simulink model "CurtisEnable"  (R2024a)
settings: Solver=FixedStepAuto  StartTime=0.0  StopTime=20  RelTol=1e-3
model workspace (MAT data in the model file):
  mdlWSDbList = ["tramontina_database_curtis.dbc" "tramontina_database_curtis_mesa.dbc"]
undefined symbols (not defined in the file): Down, Pull
libraries: tramontina_database_curtislib x5, tramontina_database_curtis_mesalib x4, speedgoatlib_IO60X_IO69X x3, speedgoatlib_IO691 x1
settings Model: Creator=anderson.bordin  LastModifiedBy=matlab.cut
settings SolverCC: ConcurrentTasks=on  PositivePriorityOrder=on
settings OptimizationCC: BlockReduction=off  OptimizeBlockIOStorage=off  EnhancedBackFolding=on  PassReuseOutputArgsThreshold=0  MaxStackSize=64  OptimizeBlockOrder=speed  DifferentSizesBufferReuse=on
settings DebuggingCC: TasksWithSamePriorityMsg=none  ParameterTunabilityLossMsg=error
settings HardwareCC: ProdBitPerLong=64  ProdLongLongMode=on  ProdHWDeviceType=Intel->x86-64 (Linux 64)
settings SFSimCC: MATLABDynamicMemAlloc=off
settings RTWCC: Description=Speedgoat Real-Time Target Machine  SystemTargetFile=speedgoat.tlc  TemplateMakefile=slrealtime_default_tmf  Toolchain=Simulink Real-Time Toolchain  BuildConfiguration=Faster Runs  CodeExecutionProfiling=on  TargetLang=C++
settings CodeAppCC: ForceParamTrailComments=on  OperatorAnnotations=on
settings SimulinkRealTimeTargetCC: InstructionSetFMA=off  LogToMDFFile=off

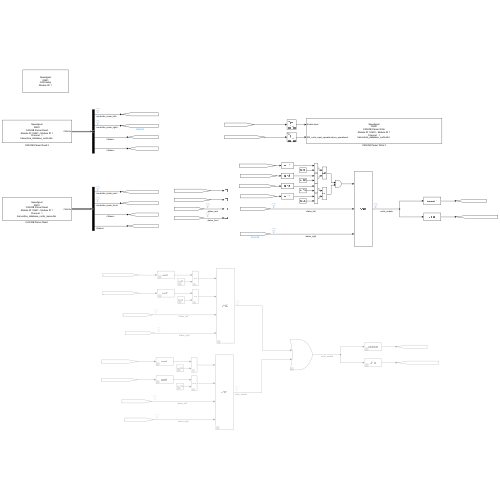
[thumbnail: Simulink's stored preview of the top-level diagram]
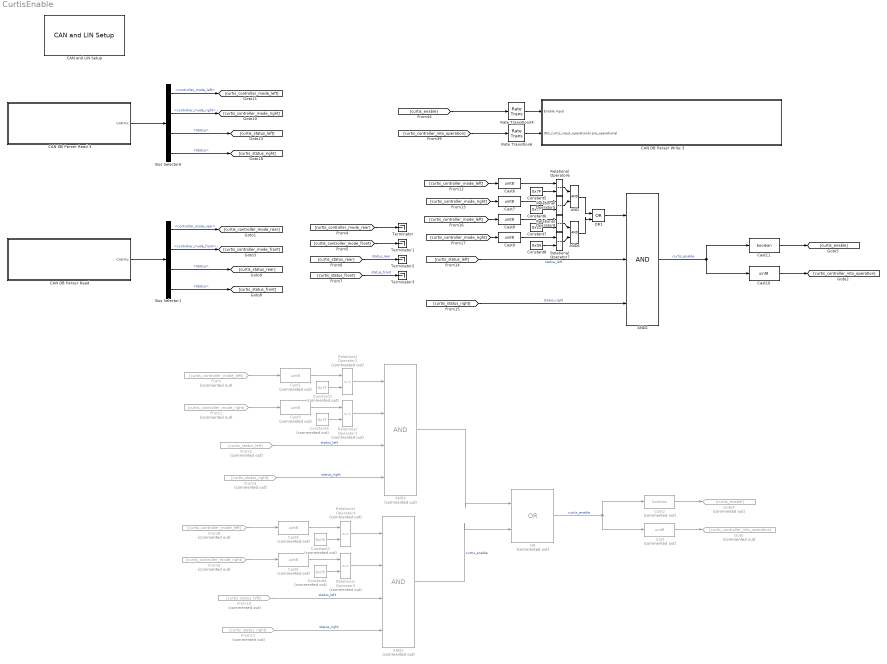
== system CurtisEnable ==
  AND : Logic  AllPortsSameDT=off  OutDataTypeStr=boolean
  AND1 : Logic  Commented=on  Inputs=4  AllPortsSameDT=off  OutDataTypeStr=boolean
  AND2 : Logic  Inputs=3  AllPortsSameDT=off  OutDataTypeStr=boolean
  AND3 : Logic  Commented=on  Inputs=4  AllPortsSameDT=off  OutDataTypeStr=boolean
  AND4 : Logic  AllPortsSameDT=off  OutDataTypeStr=boolean
  Bus Selector1 : BusSelector  OutputSignals=ID1833_controller_status_RCUrear.controller_mode_rear,ID1832_controller_status_RCUfront.controller_mode_front,ID425_curtis_feedback_message_RCUrear.MessageStatus.Status,ID424_curtis_feedback_message_RCUfront.MessageStatus.Status
  Bus Selector6 : BusSelector  OutputSignals=ID1830_controller_status_left.controller_mode_left,ID1831_controller_status_right.controller_mode_right,ID1830_controller_status_left.MessageStatus.Status,ID1831_controller_status_right.MessageStatus.Status
  "CAN DB Parser Read " : Subsystem
      settings: OpenFcn=sg_can.OpenFcnRead;
      mask Help: eval('sg.utils.help.show(''io_main/refentry_ref_can_ofa_parsing_read'');')
      mask Display: disp('Speedgoat\nIO691\nCAN DB Parser Read\nModule ID: IO691 - Module ID 1\nChannel:  1\ntramontina_database_curtis_mesa.dbc ');
  CAN DB Parser Read 3 : Subsystem
      settings: OpenFcn=sg_can.OpenFcnRead;
      mask Help: eval('sg.utils.help.show(''io_main/refentry_ref_can_ofa_parsing_read'');')
      mask Display: disp('Speedgoat\nIO691\nCAN DB Parser Read\nModule ID: IO691 - Module ID 1\nChannel:  1\ntramontina_database_curtis.dbc ');
  CAN DB Parser Write 3 : Subsystem
      settings: OpenFcn=sg_can.OpenFcnWrite;
      mask Help: eval('sg.utils.help.show(''io_main/refentry_ref_can_ofa_parsing_write'');')
      mask Display: disp('Speedgoat\nIO691\nCAN DB Parser Write\nModule ID: IO691 - Module ID 1\nChannel:  1\ntramontina_database_curtis.dbc ');
  "CAN and LIN Setup " : speedgoatlib_IO691/CAN and LIN Setup   moduleInitValues="[691    1    1   -1   -1]"  id=1  moduleType=IO691  pciSlot=-1  canChn1=CAN (HS)  canChn2=Disabled  canChn3=Disabled  canChn4=Disabled  linChn1=Disabled  linChn2=Disabled  canInitStructArray=[]  canTermStructArray=[]  gpioChnx=Disabled  canChn1InitValues="[2   2   8   1  16   3  19   2   2   5   2   0]"  arbBdrChn1=500 kBaud  clockDividerChn1=Enable  arbManBdrChn1=[8,1,16,3]  fdBdrChn1=5.0 MBaud  fdManBdrChn1=[2,2,5,2]  termResistor1=off  canChn2InitValues="[1   0   2   8  31   8  19   2   2   5   2   0]"  arbBdrChn2=1.0 MBaud  clockDividerChn2=Enable  arbManBdrChn2=[2,8,31,8]  fdBdrChn2=5.0 MBaud  fdManBdrChn2=[2,2,5,2]  termResistor2=off  canChn3InitValues="[1   0   2   8  31   8  19   2   2   5   2   0]"  arbBdrChn3=1.0 MBaud  clockDividerChn3=Enable  arbManBdrChn3=[2,8,31,8]  fdBdrChn3=5.0 MBaud  fdManBdrChn3=[2,2,5,2]  termResistor3=off  canChn4InitValues="[1   0   2   8  31   8  19   2   2   5   2   0]"  arbBdrChn4=1.0 MBaud  clockDividerChn4=Enable  arbManBdrChn4=[2,8,31,8]  fdBdrChn4=5.0 MBaud  fdManBdrChn4=[2,2,5,2]  termResistor4=off  linChn1InitValues="[0  9600]"  linBtrChn1=9600  linChn2InitValues="[0  9600]"  linBtrChn2=9600  doInitTermStruct="[0  5  0  0  0]"  parDoChannels=[1 2]  parDoVoltage=5  parDoInitValues=0  parDoReset=1  parNumOfDoS=0  parDiChannels=[3 4]  parDiVoltage=5  parDiPull=Pull-Down
      settings: LibrarySourceBlock=speedgoatlib_IO602_IO691/CAN and LIN Setup
  Cast{,1,3..5} (5 alike) : DataTypeConversion  Commented=on  OutDataTypeStr=uint8  SaturateOnIntegerOverflow=off  RndMeth=Floor
  Cast{6..10} (5 alike) : DataTypeConversion  OutDataTypeStr=uint8  SaturateOnIntegerOverflow=off  RndMeth=Floor
  Cast11 : DataTypeConversion  OutDataTypeStr=boolean  SaturateOnIntegerOverflow=off  RndMeth=Floor
  Cast2 : DataTypeConversion  Commented=on  OutDataTypeStr=boolean  SaturateOnIntegerOverflow=off  RndMeth=Floor
  Constant1 : Constant  Commented=on  Value=0x05
  Constant2 : Constant  Commented=on  Value=0x7F
  Constant3 : Constant  Commented=on  Value=0x7F
  Constant4 : Constant  Commented=on  Value=0x05
  Constant5 : Constant  Value=0x7F
  Constant6 : Constant  Value=0x7F
  Constant7 : Constant  Value=0x05
  Constant8 : Constant  Value=0x05
  From : From  Commented=on  GotoTag=curtis_controller_mode_left
  From1 : From  Commented=on  GotoTag=curtis_controller_mode_right
  From10 : From  Commented=on  GotoTag=curtis_status_left
  From11 : From  Commented=on  GotoTag=curtis_status_right
  From2 : From  Commented=on  GotoTag=curtis_status_left
  From3 : From  Commented=on  GotoTag=curtis_status_right
  From8 : From  Commented=on  GotoTag=curtis_controller_mode_left
  From9 : From  Commented=on  GotoTag=curtis_controller_mode_right
  Goto : Goto  Commented=on  GotoTag=curtis_controller_into_operation
  Goto4 : Goto  Commented=on  GotoTag=curtis_enable
  OR : Logic  Commented=on  Operator=OR  IconShape=distinctive  AllPortsSameDT=off  OutDataTypeStr=boolean
  OR1 : Logic  Operator=OR  IconShape=distinctive  AllPortsSameDT=off  OutDataTypeStr=boolean
  Rate Transition24 : RateTransition
  Rate Transition6 : RateTransition
  Relational Operator{1..4} (4 alike) : RelationalOperator  Commented=on  Operator===  OutDataTypeStr=boolean  RndMeth=Simplest  InputSameDT=off
  Relational Operator{5..8} (4 alike) : RelationalOperator  Operator===  OutDataTypeStr=boolean  RndMeth=Simplest  InputSameDT=off
  Terminator{,1..3} (4 alike) : Terminator
  wires:
  Relational Operator1/1 -> AND3/2
  From/1 -> Cast1/1
  Constant3/1 -> Relational Operator1/2
  From3/1 -> AND3/4  "status_right"
  From2/1 -> AND3/3  "status_left"
  From1/1 -> Cast3/1
  Cast/1 -> Goto/1
  Cast2/1 -> Goto4/1
  Constant2/1 -> Relational Operator2/2
  Cast3/1 -> Relational Operator1/1
  Relational Operator2/1 -> AND3/1
  Cast1/1 -> Relational Operator2/1
  Bus Selector6/1 -> [curtis_controller_mode_left]  "<controller_mode_left>"
  CAN DB Parser Read 3/1(CAN Rx) -> Bus Selector6/1
  Bus Selector6/2 -> [curtis_controller_mode_right]  "<controller_mode_right>"
  Bus Selector6/3 -> [curtis_status_left]  "<Status>"
  Bus Selector6/4 -> [curtis_status_right]  "<Status>"
  [curtis_controller_into_operation] -> Rate Transition6/1
  Rate Transition6/1 -> CAN DB Parser Write 3/2(ID0_curtis_input_operational.pre_operational)
  [curtis_enable] -> Rate Transition24/1
  Bus Selector1/1 -> [curtis_controller_mode_rear]  "<controller_mode_rear>"
  Bus Selector1/2 -> [curtis_controller_mode_front]  "<controller_mode_front>"
  "CAN DB Parser Read "/1(CAN Rx) -> Bus Selector1/1
  Bus Selector1/4 -> [curtis_status_front]  "<Status>"
  Bus Selector1/3 -> [curtis_status_rear]  "<Status>"
  [curtis_controller_mode_rear] -> Terminator/1
  [curtis_controller_mode_front] -> Terminator1/1
  [curtis_status_rear] -> Terminator2/1  "status_rear"
  [curtis_status_front] -> Terminator3/1  "status_front"
  Rate Transition24/1 -> CAN DB Parser Write 3/1(Enable Input)
  Cast4/1 -> Relational Operator4/1
  Relational Operator4/1 -> AND1/1
  Cast5/1 -> Relational Operator3/1
  Constant1/1 -> Relational Operator4/2
  From9/1 -> Cast5/1
  From10/1 -> AND1/3  "status_left"
  From11/1 -> AND1/4  "status_right"
  Constant4/1 -> Relational Operator3/2
  From8/1 -> Cast4/1
  Relational Operator3/1 -> AND1/2
  AND3/1 -> OR/1
  AND1/1 -> OR/2  "curtis_enable"
  OR/1 -> Cast/1, Cast2/1  "curtis_enable"
  Cast6/1 -> Relational Operator6/1
  Cast7/1 -> Relational Operator5/1
  Constant5/1 -> Relational Operator6/2
  [curtis_controller_mode_right] -> Cast7/1
  [curtis_status_left] -> AND2/2  "status_left"
  [curtis_status_right] -> AND2/3  "status_right"
  Constant6/1 -> Relational Operator5/2
  [curtis_controller_mode_left] -> Cast6/1
  Relational Operator6/1 -> AND/1
  Relational Operator5/1 -> AND/2
  Relational Operator7/1 -> AND4/2
  Relational Operator8/1 -> AND4/1
  [curtis_controller_mode_left] -> Cast8/1
  Constant8/1 -> Relational Operator7/2
  [curtis_controller_mode_right] -> Cast9/1
  Constant7/1 -> Relational Operator8/2
  Cast9/1 -> Relational Operator7/1
  Cast8/1 -> Relational Operator8/1
  AND/1 -> OR1/1
  AND4/1 -> OR1/2
  OR1/1 -> AND2/1
  AND2/1 -> Cast11/1, Cast10/1  "curtis_enable"
  Cast11/1 -> [curtis_enable]
  Cast10/1 -> [curtis_controller_into_operation]

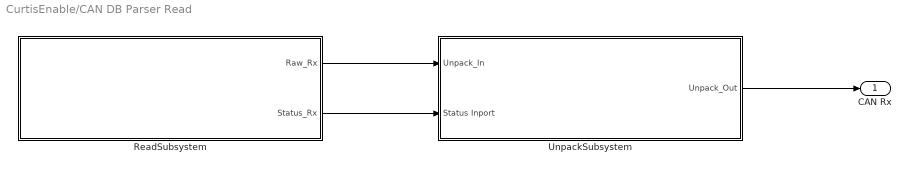
== system CurtisEnable/CAN DB Parser Read  ==
  ReadSubsystem : Subsystem
  UnpackSubsystem : Subsystem
  CAN Rx : Outport
  wires:
  ReadSubsystem/1(Raw_Rx) -> UnpackSubsystem/1(Unpack_In)
  ReadSubsystem/2(Status_Rx) -> UnpackSubsystem/2(Status Inport)
  UnpackSubsystem/1(Unpack_Out) -> CAN Rx/1

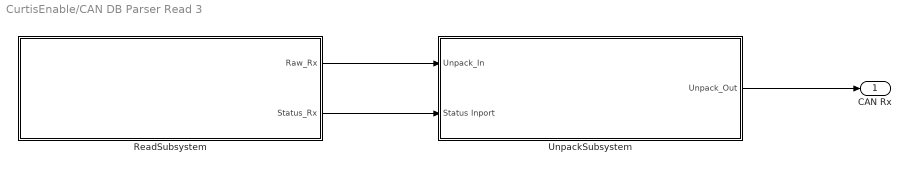
== system CurtisEnable/CAN DB Parser Read 3 ==
  ReadSubsystem : Subsystem
  UnpackSubsystem : Subsystem
  CAN Rx : Outport
  wires:
  ReadSubsystem/1(Raw_Rx) -> UnpackSubsystem/1(Unpack_In)
  ReadSubsystem/2(Status_Rx) -> UnpackSubsystem/2(Status Inport)
  UnpackSubsystem/1(Unpack_Out) -> CAN Rx/1

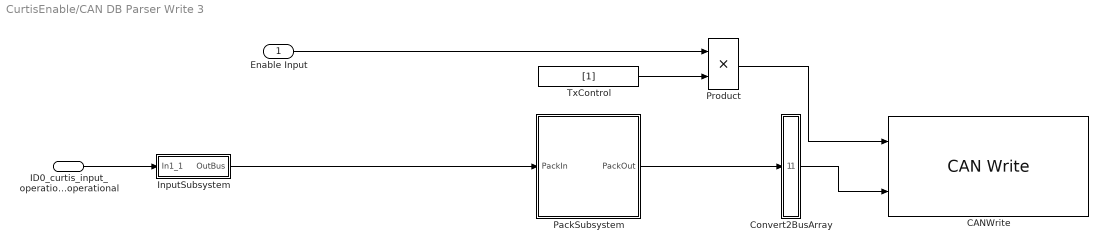
== system CurtisEnable/CAN DB Parser Write 3 ==
  Enable Input : Inport  OutDataTypeStr=boolean
  ID0_curtis_input_operational.pre_operational : Inport  Port=2
  CANWrite : speedgoatlib_IO60X_IO69X/CAN/CAN Write   moduleType=IO691  id=1  channel=1  canType=CAN (HS)  messageType=CAN (HS)  useBusIn=on  numOfMsg=1  enableInput=on  enableStatusPort=off  ts=500e-3  initValues=[691 1 0.5 0 1 1 0 1 1 1]
  Convert2BusArray : Subsystem
  InputSubsystem : Subsystem
  PackSubsystem : Subsystem
  Product : Product  OutDataTypeStr=uint32
  TxControl : Constant  Value=[1]  OutDataTypeStr=uint32
  wires:
  PackSubsystem/1(PackOut) -> Convert2BusArray/1(InBus)
  Convert2BusArray/1(BusArrayOut) -> CANWrite/2
  Product/1 -> CANWrite/1
  TxControl/1 -> Product/2
  Enable Input/1 -> Product/1
  ID0_curtis_input_operational.pre_operational/1 -> InputSubsystem/1(In1_1)
  InputSubsystem/1(OutBus) -> PackSubsystem/1(PackIn)

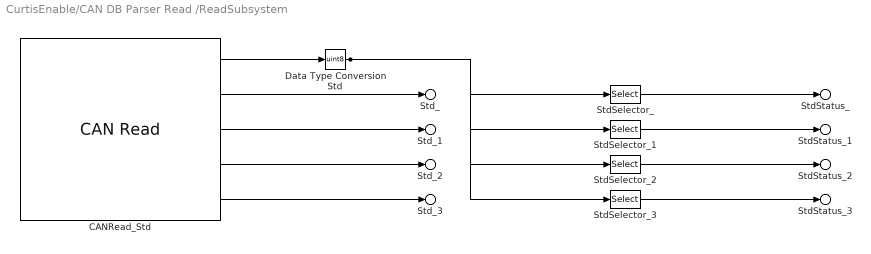
== system CurtisEnable/CAN DB Parser Read /ReadSubsystem ==
  CANRead_Std : speedgoatlib_IO60X_IO69X/CAN/CAN Read   moduleType=IO691  id=1  channel=1  canType=CAN (HS)  messageType=CAN (HS)  useBusOut=on  HasMulRead=Specify by IDs  MsgIDlist="[424   425  1832  1833]"  isEFF=off  LabelInHex=off  enableInput=off  initValues=[691 1 0.05 0 1 1 0 1 2 0 4 424 425 1832 1833]  ts=50e-3
  Data Type ConversionStd : DataTypeConversion  OutDataTypeStr=uint8  SaturateOnIntegerOverflow=off  RndMeth=Floor
  StdSelector_ : Selector  IndexOptions=Index vector (dialog)  Indices=1  OutputSizes=1
  StdSelector_1 : Selector  IndexOptions=Index vector (dialog)  Indices=2  OutputSizes=1
  StdSelector_2 : Selector  IndexOptions=Index vector (dialog)  Indices=3  OutputSizes=1
  StdSelector_3 : Selector  IndexOptions=Index vector (dialog)  Indices=4  OutputSizes=1
  Std_ : Outport  PortName=Raw_Rx  Element=Std.ID424
  Std_1 : Outport  PortName=Raw_Rx  Element=Std.ID425
  Std_2 : Outport  PortName=Raw_Rx  Element=Std.ID1832
  Std_3 : Outport  PortName=Raw_Rx  Element=Std.ID1833
  StdStatus_ : Outport  Port=2  PortName=Status_Rx  Element=Std.ID424
  StdStatus_1 : Outport  Port=2  PortName=Status_Rx  Element=Std.ID425
  StdStatus_2 : Outport  Port=2  PortName=Status_Rx  Element=Std.ID1832
  StdStatus_3 : Outport  Port=2  PortName=Status_Rx  Element=Std.ID1833
  wires:
  CANRead_Std/1 -> Data Type ConversionStd/1
  CANRead_Std/2 -> Std_/1
  CANRead_Std/3 -> Std_1/1
  CANRead_Std/4 -> Std_2/1
  CANRead_Std/5 -> Std_3/1
  Data Type ConversionStd/1 -> StdSelector_/1, StdSelector_1/1, StdSelector_2/1, StdSelector_3/1
  StdSelector_/1 -> StdStatus_/1
  StdSelector_1/1 -> StdStatus_1/1
  StdSelector_2/1 -> StdStatus_2/1
  StdSelector_3/1 -> StdStatus_3/1

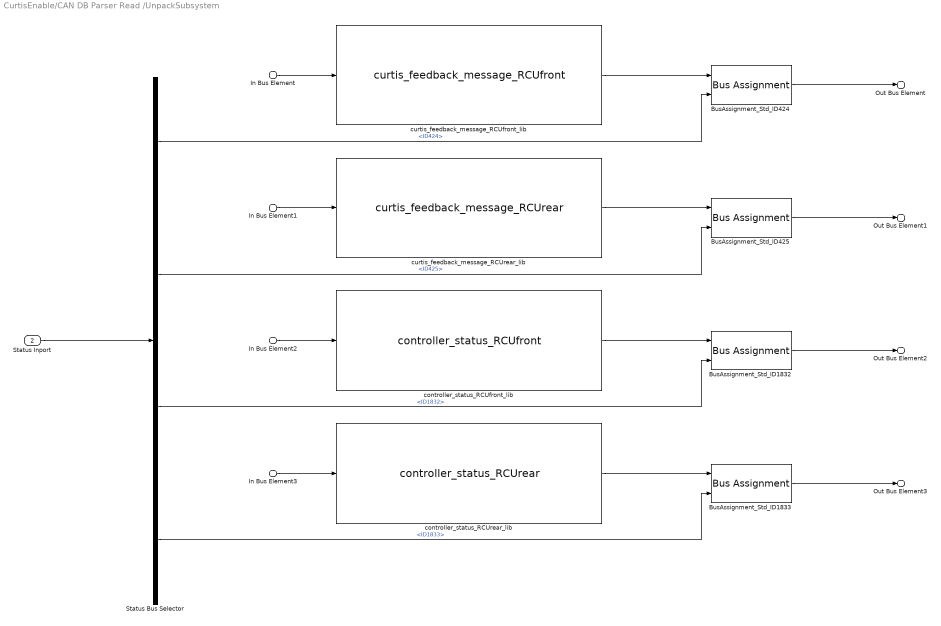
== system CurtisEnable/CAN DB Parser Read /UnpackSubsystem ==
  In Bus Element : Inport  PortName=Unpack_In  Element=Std.ID424
  In Bus Element1 : Inport  PortName=Unpack_In  Element=Std.ID425
  In Bus Element2 : Inport  PortName=Unpack_In  Element=Std.ID1832
  In Bus Element3 : Inport  PortName=Unpack_In  Element=Std.ID1833
  Status Inport : Inport  Port=2
  BusAssignment_Std_ID{424..425,1832..1833} (4 alike) : BusAssignment  AssignedSignals=MessageStatus.Status
  Status Bus Selector : BusSelector  OutputSignals=Std.ID424,Std.ID425,Std.ID1832,Std.ID1833
  controller_status_RCUfront_lib : tramontina_database_curtis_mesalib/CAN unpack/controller_status_RCUfront  SystemSampleTime=-1  VariantActivationTime=update diagram  AllowFlexibleInterface=on  Latency=0  AutoFrameSizeCalculation=off
  controller_status_RCUrear_lib : tramontina_database_curtis_mesalib/CAN unpack/controller_status_RCUrear  SystemSampleTime=-1  VariantActivationTime=update diagram  AllowFlexibleInterface=on  Latency=0  AutoFrameSizeCalculation=off
  curtis_feedback_message_RCUfront_lib : tramontina_database_curtis_mesalib/CAN unpack/curtis_feedback_message_RCUfront  SystemSampleTime=-1  VariantActivationTime=update diagram  AllowFlexibleInterface=on  Latency=0  AutoFrameSizeCalculation=off
  curtis_feedback_message_RCUrear_lib : tramontina_database_curtis_mesalib/CAN unpack/curtis_feedback_message_RCUrear  SystemSampleTime=-1  VariantActivationTime=update diagram  AllowFlexibleInterface=on  Latency=0  AutoFrameSizeCalculation=off
  Out Bus Element : Outport  PortName=Unpack_Out  Element=ID424_curtis_feedback_message_RCUfront
  Out Bus Element1 : Outport  PortName=Unpack_Out  Element=ID425_curtis_feedback_message_RCUrear
  Out Bus Element2 : Outport  PortName=Unpack_Out  Element=ID1832_controller_status_RCUfront
  Out Bus Element3 : Outport  PortName=Unpack_Out  Element=ID1833_controller_status_RCUrear
  wires:
  In Bus Element/1 -> curtis_feedback_message_RCUfront_lib/1
  curtis_feedback_message_RCUfront_lib/1 -> BusAssignment_Std_ID424/1
  BusAssignment_Std_ID424/1 -> Out Bus Element/1
  In Bus Element1/1 -> curtis_feedback_message_RCUrear_lib/1
  curtis_feedback_message_RCUrear_lib/1 -> BusAssignment_Std_ID425/1
  BusAssignment_Std_ID425/1 -> Out Bus Element1/1
  In Bus Element2/1 -> controller_status_RCUfront_lib/1
  controller_status_RCUfront_lib/1 -> BusAssignment_Std_ID1832/1
  BusAssignment_Std_ID1832/1 -> Out Bus Element2/1
  In Bus Element3/1 -> controller_status_RCUrear_lib/1
  controller_status_RCUrear_lib/1 -> BusAssignment_Std_ID1833/1
  BusAssignment_Std_ID1833/1 -> Out Bus Element3/1
  Status Inport/1 -> Status Bus Selector/1
  Status Bus Selector/1 -> BusAssignment_Std_ID424/2  "<ID424>"
  Status Bus Selector/2 -> BusAssignment_Std_ID425/2  "<ID425>"
  Status Bus Selector/3 -> BusAssignment_Std_ID1832/2  "<ID1832>"
  Status Bus Selector/4 -> BusAssignment_Std_ID1833/2  "<ID1833>"

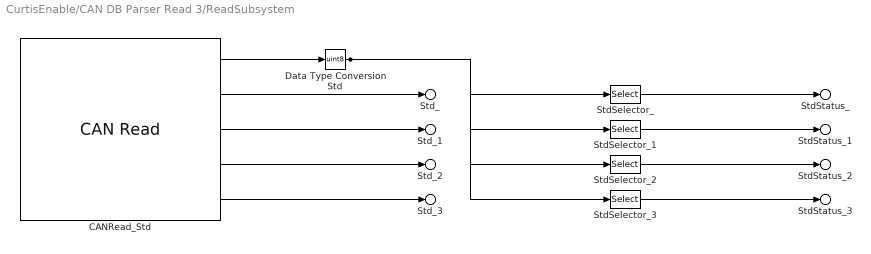
== system CurtisEnable/CAN DB Parser Read 3/ReadSubsystem ==
  CANRead_Std : speedgoatlib_IO60X_IO69X/CAN/CAN Read   moduleType=IO691  id=1  channel=1  canType=CAN (HS)  messageType=CAN (HS)  useBusOut=on  HasMulRead=Specify by IDs  MsgIDlist="[422   423  1830  1831]"  isEFF=off  LabelInHex=off  enableInput=off  initValues=[691 1 0.05 0 1 1 0 1 2 0 4 422 423 1830 1831]  ts=50e-3
  Data Type ConversionStd : DataTypeConversion  OutDataTypeStr=uint8  SaturateOnIntegerOverflow=off  RndMeth=Floor
  StdSelector_ : Selector  IndexOptions=Index vector (dialog)  Indices=1  OutputSizes=1
  StdSelector_1 : Selector  IndexOptions=Index vector (dialog)  Indices=2  OutputSizes=1
  StdSelector_2 : Selector  IndexOptions=Index vector (dialog)  Indices=3  OutputSizes=1
  StdSelector_3 : Selector  IndexOptions=Index vector (dialog)  Indices=4  OutputSizes=1
  Std_ : Outport  PortName=Raw_Rx  Element=Std.ID422
  Std_1 : Outport  PortName=Raw_Rx  Element=Std.ID423
  Std_2 : Outport  PortName=Raw_Rx  Element=Std.ID1830
  Std_3 : Outport  PortName=Raw_Rx  Element=Std.ID1831
  StdStatus_ : Outport  Port=2  PortName=Status_Rx  Element=Std.ID422
  StdStatus_1 : Outport  Port=2  PortName=Status_Rx  Element=Std.ID423
  StdStatus_2 : Outport  Port=2  PortName=Status_Rx  Element=Std.ID1830
  StdStatus_3 : Outport  Port=2  PortName=Status_Rx  Element=Std.ID1831
  wires:
  CANRead_Std/1 -> Data Type ConversionStd/1
  CANRead_Std/2 -> Std_/1
  CANRead_Std/3 -> Std_1/1
  CANRead_Std/4 -> Std_2/1
  CANRead_Std/5 -> Std_3/1
  Data Type ConversionStd/1 -> StdSelector_/1, StdSelector_1/1, StdSelector_2/1, StdSelector_3/1
  StdSelector_/1 -> StdStatus_/1
  StdSelector_1/1 -> StdStatus_1/1
  StdSelector_2/1 -> StdStatus_2/1
  StdSelector_3/1 -> StdStatus_3/1

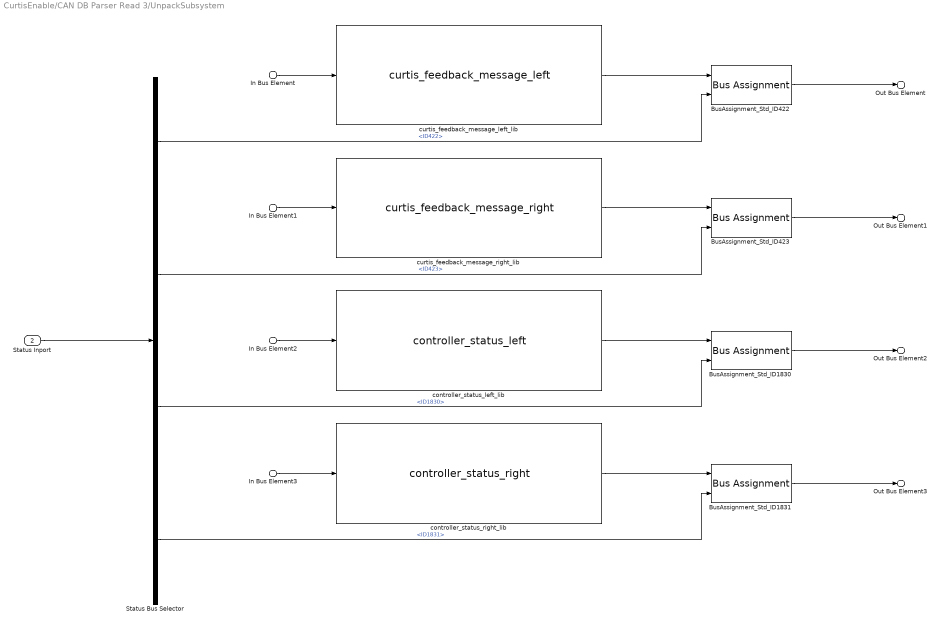
== system CurtisEnable/CAN DB Parser Read 3/UnpackSubsystem ==
  In Bus Element : Inport  PortName=Unpack_In  Element=Std.ID422
  In Bus Element1 : Inport  PortName=Unpack_In  Element=Std.ID423
  In Bus Element2 : Inport  PortName=Unpack_In  Element=Std.ID1830
  In Bus Element3 : Inport  PortName=Unpack_In  Element=Std.ID1831
  Status Inport : Inport  Port=2
  BusAssignment_Std_ID{422..423,1830..1831} (4 alike) : BusAssignment  AssignedSignals=MessageStatus.Status
  Status Bus Selector : BusSelector  OutputSignals=Std.ID422,Std.ID423,Std.ID1830,Std.ID1831
  controller_status_left_lib : tramontina_database_curtislib/CAN unpack/controller_status_left  SystemSampleTime=-1  VariantActivationTime=update diagram  AllowFlexibleInterface=on  Latency=0  AutoFrameSizeCalculation=off
  controller_status_right_lib : tramontina_database_curtislib/CAN unpack/controller_status_right  SystemSampleTime=-1  VariantActivationTime=update diagram  AllowFlexibleInterface=on  Latency=0  AutoFrameSizeCalculation=off
  curtis_feedback_message_left_lib : tramontina_database_curtislib/CAN unpack/curtis_feedback_message_left  SystemSampleTime=-1  VariantActivationTime=update diagram  AllowFlexibleInterface=on  Latency=0  AutoFrameSizeCalculation=off
  curtis_feedback_message_right_lib : tramontina_database_curtislib/CAN unpack/curtis_feedback_message_right  SystemSampleTime=-1  VariantActivationTime=update diagram  AllowFlexibleInterface=on  Latency=0  AutoFrameSizeCalculation=off
  Out Bus Element : Outport  PortName=Unpack_Out  Element=ID422_curtis_feedback_message_left
  Out Bus Element1 : Outport  PortName=Unpack_Out  Element=ID423_curtis_feedback_message_right
  Out Bus Element2 : Outport  PortName=Unpack_Out  Element=ID1830_controller_status_left
  Out Bus Element3 : Outport  PortName=Unpack_Out  Element=ID1831_controller_status_right
  wires:
  In Bus Element/1 -> curtis_feedback_message_left_lib/1
  curtis_feedback_message_left_lib/1 -> BusAssignment_Std_ID422/1
  BusAssignment_Std_ID422/1 -> Out Bus Element/1
  In Bus Element1/1 -> curtis_feedback_message_right_lib/1
  curtis_feedback_message_right_lib/1 -> BusAssignment_Std_ID423/1
  BusAssignment_Std_ID423/1 -> Out Bus Element1/1
  In Bus Element2/1 -> controller_status_left_lib/1
  controller_status_left_lib/1 -> BusAssignment_Std_ID1830/1
  BusAssignment_Std_ID1830/1 -> Out Bus Element2/1
  In Bus Element3/1 -> controller_status_right_lib/1
  controller_status_right_lib/1 -> BusAssignment_Std_ID1831/1
  BusAssignment_Std_ID1831/1 -> Out Bus Element3/1
  Status Inport/1 -> Status Bus Selector/1
  Status Bus Selector/1 -> BusAssignment_Std_ID422/2  "<ID422>"
  Status Bus Selector/2 -> BusAssignment_Std_ID423/2  "<ID423>"
  Status Bus Selector/3 -> BusAssignment_Std_ID1830/2  "<ID1830>"
  Status Bus Selector/4 -> BusAssignment_Std_ID1831/2  "<ID1831>"

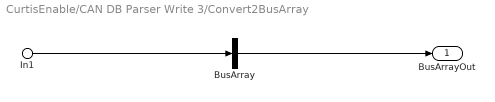
== system CurtisEnable/CAN DB Parser Write 3/Convert2BusArray ==
  In1 : Inport  PortName=InBus  Element=ID0_curtis_input_operational
  BusArray : Concatenate  NumInputs=1
  BusArrayOut : Outport
  wires:
  In1/1 -> BusArray/1
  BusArray/1 -> BusArrayOut/1

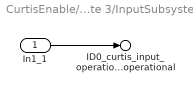
== system CurtisEnable/CAN DB Parser Write 3/InputSubsystem ==
  In1_1 : Inport
  ID0_curtis_input_operational.pre_operational : Outport  PortName=OutBus  Element=ID0_curtis_input_operational.pre_operational
  wires:
  In1_1/1 -> ID0_curtis_input_operational.pre_operational/1

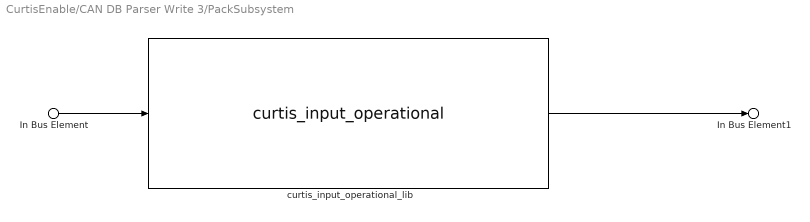
== system CurtisEnable/CAN DB Parser Write 3/PackSubsystem ==
  In Bus Element : Inport  PortName=PackIn  Element=ID0_curtis_input_operational
  curtis_input_operational_lib : tramontina_database_curtislib/CAN pack/curtis_input_operational  SystemSampleTime=-1  VariantActivationTime=update diagram  AllowFlexibleInterface=on  Latency=0  AutoFrameSizeCalculation=off
  In Bus Element1 : Outport  PortName=PackOut  Element=ID0_curtis_input_operational
  wires:
  In Bus Element/1 -> curtis_input_operational_lib/1
  curtis_input_operational_lib/1 -> In Bus Element1/1
